simulink model "StatesComparison"  (R2018a)
settings: Solver=VariableStepAuto  StartTime=0.0  StopTime=10.0  RelTol=1e-3
PreLoadFcn:
  | modelDir = fileparts(get_param(bdroot, 'FileName'));
  | addpath(fullfile(modelDir,'../../Misc'));
settings Model: Creator=Thomas  LastModifiedBy=Thomas

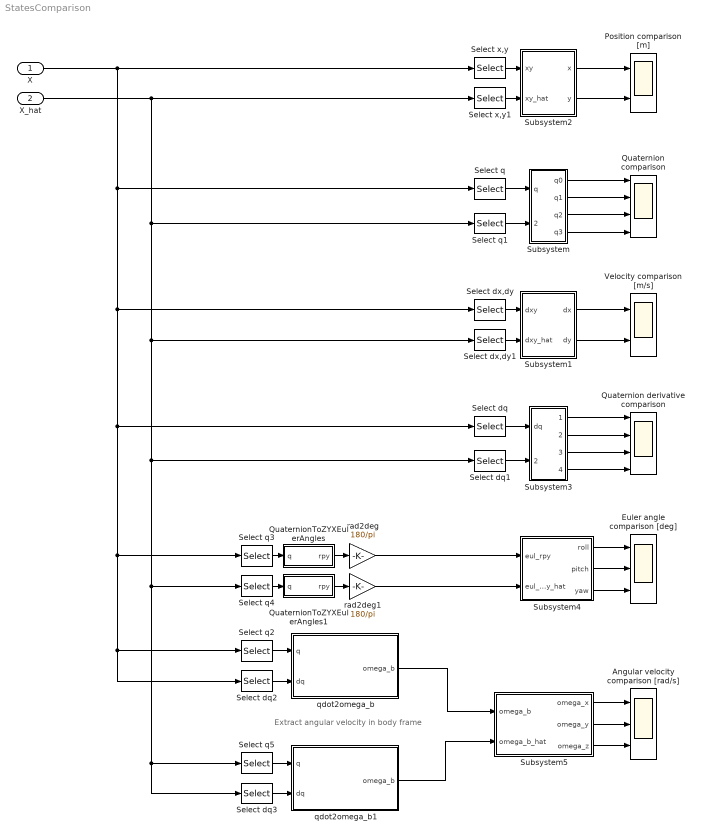
== system StatesComparison ==
  note: Extract angular velocity in body frame
  X : Inport
  X_hat : Inport  Port=2
  Angular velocity comparison [rad/s] : Scope  NumInputPorts=3
  Euler angle comparison [deg] : Scope  NumInputPorts=3
  Position comparison [m] : Scope  NumInputPorts=2
  Quaternion comparison : Scope  NumInputPorts=4
  Quaternion derivative comparison : Scope  NumInputPorts=4
  QuaternionToZYXEulerAngles : MATLAB Function  TreatAsAtomicUnit=on
  QuaternionToZYXEulerAngles1 : MATLAB Function  TreatAsAtomicUnit=on
  Select dq{,1..3} (4 alike) : Selector  InputPortWidth=12  IndexOptions=Index vector (dialog)  Indices=[9,10,11,12]  OutputSizes=1
  Select dx,dy : Selector  InputPortWidth=12  IndexOptions=Index vector (dialog)  Indices=[7,8]  OutputSizes=1
  Select dx,dy1 : Selector  InputPortWidth=12  IndexOptions=Index vector (dialog)  Indices=[7,8]  OutputSizes=1
  Select q{,1..5} (6 alike) : Selector  InputPortWidth=12  IndexOptions=Index vector (dialog)  Indices=[3,4,5,6]  OutputSizes=1
  Select x,y : Selector  InputPortWidth=12  IndexOptions=Index vector (dialog)  Indices=[1,2]  OutputSizes=1
  Select x,y1 : Selector  InputPortWidth=12  IndexOptions=Index vector (dialog)  Indices=[1,2]  OutputSizes=1
  Subsystem : Subsystem
  Subsystem1 : Subsystem
  Subsystem2 : Subsystem
  Subsystem3 : Subsystem
  Subsystem4 : Subsystem
  Subsystem5 : Subsystem
  Velocity comparison [m/s] : Scope  NumInputPorts=2
  qdot2omega_b : MATLAB Function  TreatAsAtomicUnit=on
  qdot2omega_b1 : MATLAB Function  TreatAsAtomicUnit=on
  rad2deg : Gain  Gain=180/pi
  rad2deg1 : Gain  Gain=180/pi
  wires:
  Subsystem/2(q1) -> Quaternion comparison/2
  Subsystem/4(q3) -> Quaternion comparison/4
  Subsystem/3(q2) -> Quaternion comparison/3
  Subsystem/1(q0) -> Quaternion comparison/1
  Subsystem1/1(dx) -> Velocity comparison [m/s]/1
  Subsystem1/2(dy) -> Velocity comparison [m/s]/2
  Select q1/1 -> Subsystem/2(q_hat)
  Select q/1 -> Subsystem/1(q)
  X_hat/1 -> Select q1/1, Select dq3/1, Select q5/1, Select q4/1, Select dq1/1, Select dx,dy1/1, Select x,y1/1
  Select dx,dy/1 -> Subsystem1/1(dxy)
  Select dx,dy1/1 -> Subsystem1/2(dxy_hat)
  Subsystem2/1(x) -> Position comparison [m]/1
  Subsystem2/2(y) -> Position comparison [m]/2
  Select x,y/1 -> Subsystem2/1(xy)
  Select x,y1/1 -> Subsystem2/2(xy_hat)
  Subsystem3/1(dq0) -> Quaternion derivative comparison/1
  Subsystem3/4(dq3) -> Quaternion derivative comparison/4
  Subsystem3/3(dq2) -> Quaternion derivative comparison/3
  Subsystem3/2(dq1) -> Quaternion derivative comparison/2
  Select dq/1 -> Subsystem3/1(dq)
  Select dq1/1 -> Subsystem3/2(dq_hat)
  Select q2/1 -> qdot2omega_b/1(q)
  Select dq2/1 -> qdot2omega_b/2(dq)
  Select q3/1 -> QuaternionToZYXEulerAngles/1(q)
  Select q4/1 -> QuaternionToZYXEulerAngles1/1(q)
  QuaternionToZYXEulerAngles1/1(rpy) -> rad2deg1/1
  QuaternionToZYXEulerAngles/1(rpy) -> rad2deg/1
  rad2deg/1 -> Subsystem4/1(eul_rpy)
  rad2deg1/1 -> Subsystem4/2(eul_rpy_hat)
  Subsystem4/1(roll) -> Euler angle comparison [deg]/1
  Subsystem4/2(pitch) -> Euler angle comparison [deg]/2
  Subsystem4/3(yaw) -> Euler angle comparison [deg]/3
  Select q5/1 -> qdot2omega_b1/1(q)
  Select dq3/1 -> qdot2omega_b1/2(dq)
  X/1 -> Select dq2/1, Select q2/1, Select q3/1, Select dq/1, Select dx,dy/1, Select q/1, Select x,y/1
  Subsystem5/1(omega_x) -> Angular velocity comparison [rad/s]/1
  Subsystem5/2(omega_y) -> Angular velocity comparison [rad/s]/2
  Subsystem5/3(omega_z) -> Angular velocity comparison [rad/s]/3
  qdot2omega_b/1(omega_b) -> Subsystem5/1(omega_b)
  qdot2omega_b1/1(omega_b) -> Subsystem5/2(omega_b_hat)

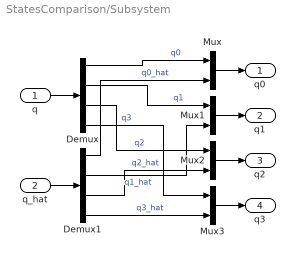
== system StatesComparison/Subsystem ==
  q : Inport
  q_hat : Inport  Port=2
  Demux : Demux
  Demux1 : Demux
  Mux{,1..3} (4 alike) : Mux  Inputs=2
  q0 : Outport
  q1 : Outport  Port=2
  q2 : Outport  Port=3
  q3 : Outport  Port=4
  wires:
  Demux1/2 -> Mux1/2  "q1_hat"
  Demux1/3 -> Mux2/2  "q2_hat"
  Demux/4 -> Mux3/1  "q3"
  Mux1/1 -> q1/1
  Demux1/4 -> Mux3/2  "q3_hat"
  Demux/3 -> Mux2/1  "q2"
  Demux1/1 -> Mux/2  "q0_hat"
  Mux2/1 -> q2/1
  q_hat/1 -> Demux1/1
  Demux/1 -> Mux/1  "q0"
  Mux/1 -> q0/1
  Demux/2 -> Mux1/1  "q1"
  q/1 -> Demux/1
  Mux3/1 -> q3/1

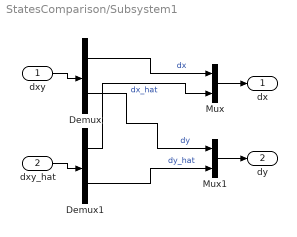
== system StatesComparison/Subsystem1 ==
  dxy : Inport
  dxy_hat : Inport  Port=2
  Demux : Demux  Outputs=2
  Demux1 : Demux  Outputs=2
  Mux : Mux  Inputs=2
  Mux1 : Mux  Inputs=2
  dx : Outport
  dy : Outport  Port=2
  wires:
  Demux1/2 -> Mux1/2  "dy_hat"
  Mux1/1 -> dy/1
  Demux1/1 -> Mux/2  "dx_hat"
  dxy_hat/1 -> Demux1/1
  Demux/1 -> Mux/1  "dx"
  Mux/1 -> dx/1
  Demux/2 -> Mux1/1  "dy"
  dxy/1 -> Demux/1

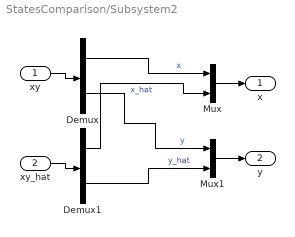
== system StatesComparison/Subsystem2 ==
  xy : Inport
  xy_hat : Inport  Port=2
  Demux : Demux  Outputs=2
  Demux1 : Demux  Outputs=2
  Mux : Mux  Inputs=2
  Mux1 : Mux  Inputs=2
  x : Outport
  y : Outport  Port=2
  wires:
  Demux1/2 -> Mux1/2  "y_hat"
  Mux1/1 -> y/1
  Demux1/1 -> Mux/2  "x_hat"
  xy_hat/1 -> Demux1/1
  Demux/1 -> Mux/1  "x"
  Mux/1 -> x/1
  Demux/2 -> Mux1/1  "y"
  xy/1 -> Demux/1

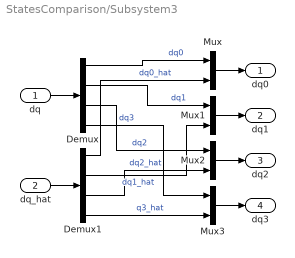
== system StatesComparison/Subsystem3 ==
  dq : Inport
  dq_hat : Inport  Port=2
  Demux : Demux
  Demux1 : Demux
  Mux{,1..3} (4 alike) : Mux  Inputs=2
  dq0 : Outport
  dq1 : Outport  Port=2
  dq2 : Outport  Port=3
  dq3 : Outport  Port=4
  wires:
  Demux1/2 -> Mux1/2  "dq1_hat"
  Demux1/3 -> Mux2/2  "dq2_hat"
  Demux/4 -> Mux3/1  "dq3"
  Mux1/1 -> dq1/1
  Demux1/4 -> Mux3/2  "q3_hat"
  Demux/3 -> Mux2/1  "dq2"
  Demux1/1 -> Mux/2  "dq0_hat"
  Mux2/1 -> dq2/1
  dq_hat/1 -> Demux1/1
  Demux/1 -> Mux/1  "dq0"
  Mux/1 -> dq0/1
  Demux/2 -> Mux1/1  "dq1"
  dq/1 -> Demux/1
  Mux3/1 -> dq3/1

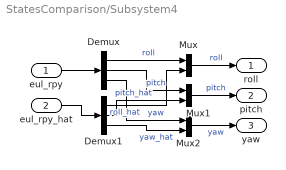
== system StatesComparison/Subsystem4 ==
  eul_rpy : Inport
  eul_rpy_hat : Inport  Port=2
  Demux : Demux  Outputs=3
  Demux1 : Demux  Outputs=3
  Mux : Mux  Inputs=2
  Mux1 : Mux  Inputs=2
  Mux2 : Mux  Inputs=2
  roll : Outport
  pitch : Outport  Port=2
  yaw : Outport  Port=3
  wires:
  Demux/2 -> Mux1/1  "pitch"
  Demux/1 -> Mux/1  "roll"
  Mux/1 -> roll/1  "roll"
  Demux/3 -> Mux2/1  "yaw"
  Demux1/3 -> Mux2/2  "yaw_hat"
  eul_rpy/1 -> Demux/1
  Demux1/1 -> Mux/2  "roll_hat"
  Demux1/2 -> Mux1/2  "pitch_hat"
  Mux2/1 -> yaw/1  "yaw"
  eul_rpy_hat/1 -> Demux1/1
  Mux1/1 -> pitch/1  "pitch"

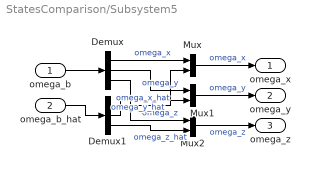
== system StatesComparison/Subsystem5 ==
  omega_b : Inport
  omega_b_hat : Inport  Port=2
  Demux : Demux  Outputs=3
  Demux1 : Demux  Outputs=3
  Mux : Mux  Inputs=2
  Mux1 : Mux  Inputs=2
  Mux2 : Mux  Inputs=2
  omega_x : Outport
  omega_y : Outport  Port=2
  omega_z : Outport  Port=3
  wires:
  Demux/2 -> Mux1/1  "omega_y"
  Demux/1 -> Mux/1  "omega_x"
  Mux/1 -> omega_x/1  "omega_x"
  Demux/3 -> Mux2/1  "omega_z"
  Demux1/3 -> Mux2/2  "omega_z_hat"
  omega_b/1 -> Demux/1
  Demux1/1 -> Mux/2  "omega_x_hat"
  Demux1/2 -> Mux1/2  "omega_y_hat"
  Mux2/1 -> omega_z/1  "omega_z"
  omega_b_hat/1 -> Demux1/1
  Mux1/1 -> omega_y/1  "omega_y"

== matlab function StatesComparison/QuaternionToZYXEulerAngles ==
  data: q input; rpy output
function rpy = Quaternion2ZYXEulerAngles(q)
    rpy = Quaternion2ZYXEulerAngles(q);
end

== matlab function StatesComparison/QuaternionToZYXEulerAngles1 ==
  data: q input; rpy output
function rpy = Quaternion2ZYXEulerAngles(q)
    rpy = Quaternion2ZYXEulerAngles(q);
end

== matlab function StatesComparison/qdot2omega_b ==
  data: q input; omega_b output; dq input
function omega_b = qdot2omega_b(q, dq)
    omega_b = qdot2omega_b(q, dq);
end

== matlab function StatesComparison/qdot2omega_b1 ==
  data: q input; omega_b output; dq input
function omega_b = qdot2omega_b(q, dq)
    omega_b = qdot2omega_b(q, dq);
end
